simulink model "rigid_comp"  (R2022a)
settings: Solver=FixedStepAuto  StartTime=0.0  StopTime=Sim_time  FixedStep=.001  RelTol=1e-3
values from neighbouring files (symbols this model uses):
  Amplitude = 0.2    [flexible_main.m]    (also in rigid_main.m = 0.5)
  B = .05    (= 0.05)    [parameters.m]
  dead_zone = 0.25    [flexible_main.m]    (also in rigid_main.m = 0.7)
  Frequency = 0.1    [flexible_main.m]    (also in rigid_main.m = 0.2)
  J = J_hub + J_load + J_extra    (= 0.017612872)    [parameters.m]
  Kdd = 0    [flexible_main.m]    (also in rigid_main.m)
  Kdt = 0    [flexible_main.m]    (also in rigid_main.m = 0.5)
  Kg = 33.3    [parameters.m]
  Km = 0.0401    [parameters.m]
  Kpd = 0    [flexible_main.m]    (also in rigid_main.m)
  Kpt = 15    [flexible_main.m]    (also in rigid_main.m = 10.5)
  Rm = 19.2    [parameters.m]
  saturation = 10    [flexible_main.m]    (also in rigid_main.m)
libraries: vrlib x3, simulink x1
settings Model: Creator=bobbyhodgkinson  LastModifiedBy=hodgkinr
settings SolverCC: AlgebraicLoopSolver=TrustRegion
settings DebuggingCC: UnconnectedInputMsg=warning  UnconnectedOutputMsg=warning  UnconnectedLineMsg=warning  SFMachineParentedDataDiag=warning  ArithmeticOperatorsInVariantConditions=warning
settings SFSimCC: CustomCodeUndefinedFunction=UseInterfaceOnly
settings CodeAppCC: StateflowObjectComments=on

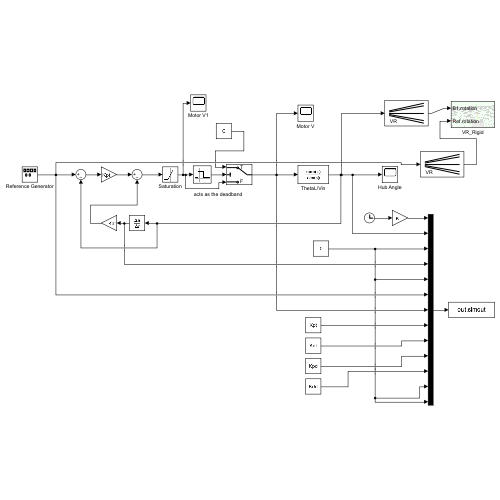
[thumbnail: Simulink's stored preview of the top-level diagram]
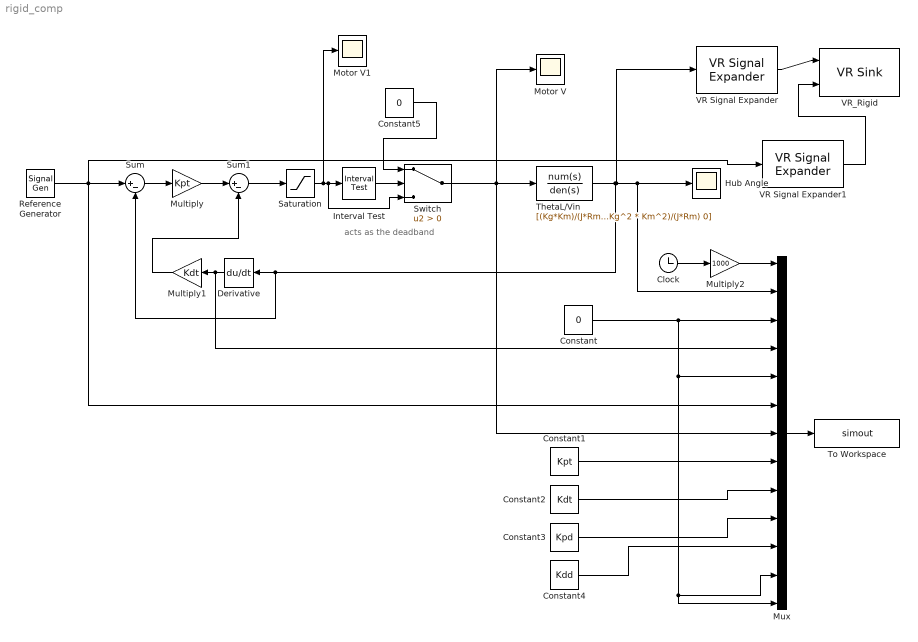
== system rigid_comp ==
  note: acts as the deadband
  Clock : Clock
  Constant : Constant  Value=0
  Constant1 : Constant  Value=Kpt
  Constant2 : Constant  Value=Kdt
  Constant3 : Constant  Value=Kpd
  Constant4 : Constant  Value=Kdd
  Constant5 : Constant  Value=0
  Derivative : Derivative  CoefficientInTFapproximation=0
  Hub Angle : Scope
  Interval Test : simulink/Logic and Bit Operations/Interval Test  IntervalClosedRight=on  uplimit=dead_zone  IntervalClosedLeft=on  lowlimit=-1*dead_zone  OutDataTypeStr=boolean
  Motor V : Scope
  Motor V1 : Scope
  Multiply : Gain  Gain=Kpt
  Multiply1 : Gain  Gain=Kdt
  Multiply2 : Gain  Gain=1000
  Mux : Mux  Inputs=13
  Reference Generator : SignalGenerator  WaveForm=square  Amplitude=Amplitude  Frequency=Frequency
  Saturation : Saturate  UpperLimit=saturation  LowerLimit=-1*saturation
  Sum : Sum  Inputs=|+-
  Sum1 : Sum  Inputs=|+-
  Switch : Switch  Criteria=u2 > Threshold  SaturateOnIntegerOverflow=off  InputSameDT=off
  "ThetaL/Vin " : TransferFcn  Numerator=[(Kg*Km)/(J*Rm)]  Denominator=[1 (B/J)+(Kg^2 * Km^2)/(J*Rm) 0]
  To Workspace : ToWorkspace  VariableName=simout  SaveFormat=Timeseries  SampleTime=-1
  VR Signal Expander : vrlib/VR Signal Expander  outwidth=4  outidx=[4]
  VR Signal Expander1 : vrlib/VR Signal Expander  outwidth=4  outidx=[4]
  VR_Rigid : vrlib/VR Sink  InstantiateOnLoad=on  SampleTime=0.01  ViewEnable=on  RemoteChange=off  RemoteView=off  FieldsWritten=B1.rotation.4.1.1.double#Ref.rotation.4.1.1.double  WorldFileName=rigid_2020.wrl  AutoView=off  VideoDimensions=[]  AllowVariableSize=off
  wires:
  Reference Generator/1 -> VR Signal Expander1/1, Sum/1, Mux/6
  Sum/1 -> Multiply/1
  Multiply/1 -> Sum1/1
  "ThetaL/Vin "/1 -> VR Signal Expander/1, Mux/2, Hub Angle/1, Sum/2, Derivative/1
  Derivative/1 -> Mux/4, Multiply1/1
  Multiply1/1 -> Sum1/2
  Sum1/1 -> Saturation/1
  Saturation/1 -> Switch/3, Interval Test/1, Motor V1/1
  Switch/1 -> Mux/7, "ThetaL/Vin "/1, Motor V/1
  Mux/1 -> To Workspace/1
  Constant/1 -> Mux/13, Mux/12, Mux/5, Mux/3
  Constant1/1 -> Mux/8
  Constant2/1 -> Mux/9
  Constant3/1 -> Mux/10
  Constant4/1 -> Mux/11
  Clock/1 -> Multiply2/1
  Multiply2/1 -> Mux/1
  VR Signal Expander/1 -> VR_Rigid/1
  VR Signal Expander1/1 -> VR_Rigid/2
  Interval Test/1 -> Switch/2
  Constant5/1 -> Switch/1
